simulink model "QPSK_complete2"  (R2016b)
settings: Solver=VariableStepAuto  StartTime=0.0  StopTime=(12+226)*8  RelTol=1e-3  EnableMultiTasking=on
undefined symbols (not defined in the file or in its folder): jsin, K1, K2, rcosine
libraries: dspsigops x2, dspstat3 x1, dspsrcs4 x1, simulink x1
settings Model: Creator=coltmt  LastModifiedBy=colttom
settings OptimizationCC: LifeSpan=inf
settings DebuggingCC: SFUnexpectedBacktrackingDiag=warning  SFNoUnconditionalDefaultTransitionDiag=warning  SFExecutionAtInitializationDiag=none
settings GRTTargetCC: TargetLangStandard=C89/C90 (ANSI)  GeneratePreprocessorConditionals=Disable all
settings ConfigComp: CovMetricSettings=dw  CovHtmlReporting=on  CovSaveCumulativeToWorkspaceVar=on  CovSaveSingleToWorkspaceVar=on  CovExternalEMLEnable=off

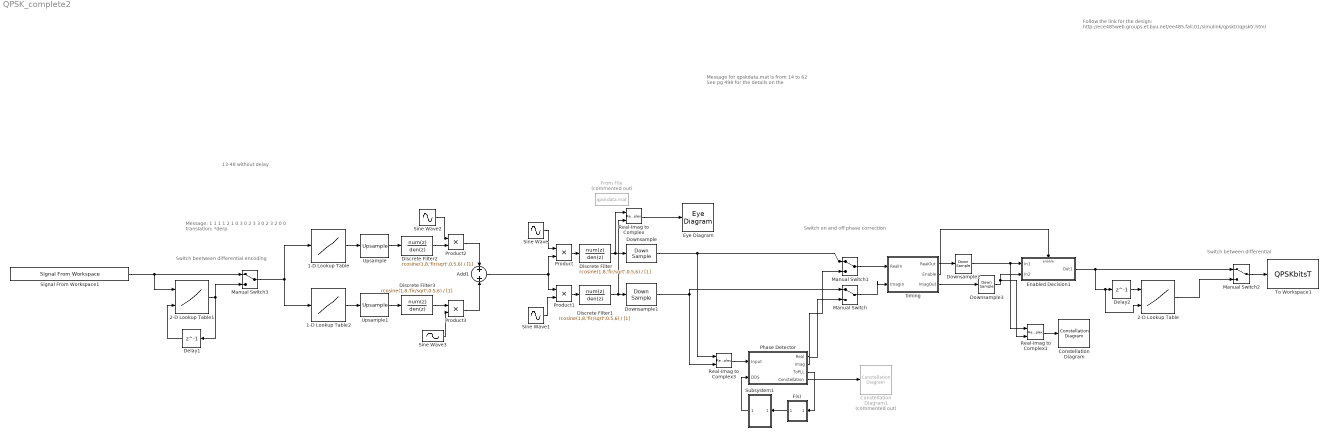
== system QPSK_complete2 ==
  note: Switch beetween differential encoding
  note: Switch between differential
  note: Switch on and off phase correction
  note: 13-48 without delay
  note: Message: 1 1 1 1 2 1 0 3 0 2 3 3 0 2 3 2 0 0
      | translation: *derp
  note: Follow the link for the design: http://ece485web.groups.et.byu.net/ee485.fall.01/simulink/qpsktr/qpsktr.html
  note: Message for qpskdata.mat is from 14 to 62
      |
      | See pg 498 for the details on the
  1-D Lookup Table : Lookup_n-D  NumberOfTableDimensions=1  BreakpointsForDimension1=[0 1 2 3]  Table=[1 -1 1 -1]*3/sqrt(2)  InternalRulePriority=Speed  RndMeth=Simplest  InputSameDT=on
  1-D Lookup Table2 : Lookup_n-D  NumberOfTableDimensions=1  BreakpointsForDimension1=[0 1 2 3]  Table=[1 1 -1 -1]*3/sqrt(2)  InternalRulePriority=Speed  RndMeth=Simplest  InputSameDT=on
  2-D Lookup Table : Lookup_n-D  BreakpointsForDimension1=[0:3]  BreakpointsForDimension2=[0:3]  Table=[0 1 2 3; 2 0 3 1; 1 3 0 2;3 2 1 0]  InternalRulePriority=Speed  RndMeth=Simplest  InputSameDT=on
  2-D Lookup Table1 : Lookup_n-D  BreakpointsForDimension1=[0:3]  BreakpointsForDimension2=[0:3]  Table=[0 1 2 3;1 3 0 2;2 0 3 1;3 2 1 0]  InternalRulePriority=Speed  RndMeth=Simplest  InputSameDT=on
  Add1 : Sum
  Constellation Diagram : ConstellationDiagram
  Constellation Diagram1 : ConstellationDiagram  Commented=on
  Delay1 : Delay  DelayLength=1
  Delay2 : Delay  DelayLength=1
  Discrete Filter{,1..3} (4 alike) : DiscreteFilter  Numerator=rcosine(1,8,'fir/sqrt',0.5,6)  Denominator=[1]
  Downsample : DownSample  N=16/2  InputProcessing=Inherited (this choice will be removed - see release notes)  RateOptions=Allow multirate processing
  Downsample1 : DownSample  N=16/2  InputProcessing=Inherited (this choice will be removed - see release notes)  RateOptions=Allow multirate processing
  Downsample2 : DownSample  RateOptions=Allow multirate processing
  Downsample3 : DownSample  RateOptions=Allow multirate processing
  Enabled Decision1 : Subsystem  TreatAsAtomicUnit=on
  Eye Diagram : EyeDiagram
  F(s) : Subsystem
  From File : FromFile  Commented=on  FileName=qpskdata.mat  SampleTime=1
  Manual Switch{,1..3} (4 alike) : ManualSwitch
  Phase Detector : Subsystem
  Product{,1..3} (4 alike) : Product
  Real-Imag to Complex : RealImagToComplex
  Real-Imag to Complex1 : RealImagToComplex
  Real-Imag to Complex3 : RealImagToComplex
  Signal From Workspace1 : dspsrcs4/Signal From Workspace  X=[1 2 3 0 0 2 3 1 3 2 1 0 3 2 0 2 0 1 4 2 3 1 0 2 3 1 2 3 0 3 2 1 2 3 0 2 3 3 1 2 3 1 2 3 1 2 3 1 2 1 2 1 2 2 1 2 1 2 1 2 1 2 1 2 1 2 1 2 1 2 1 0 0 3 2 0 1 2 0 1 3 2 3 1 1 1 1 1 0 0 0 1 1 0 0 1 1 1 1 2 1 0 3 0 2 3 3 0 2 3 2 0 0]  Ts=8  nsamps=1  OutputAfterFinalValue=Setting to zero  ignoreOrWarnInputAndFrameLengths=off  OutputFrames=off
  Sine Wave : Sin  Amplitude=sqrt(2)  Frequency=2*pi/4  Phase=pi/2  SampleTime=.5
  Sine Wave1 : Sin  Amplitude=-sqrt(2)  Frequency=2*pi/4  SampleTime=.5
  Sine Wave2 : Sin  Amplitude=sqrt(2)  Frequency=2*pi/4  Phase=pi/2  SampleTime=.5
  Sine Wave3 : Sin  Amplitude=-sqrt(2)  Frequency=2*pi/4  SampleTime=.5
  Subsystem1 : Subsystem
  To Workspace1 : ToWorkspace  VariableName=QPSKbitsT  SampleTime=-1
      settings: Save2DSignal=2-D array (concatenate along first dimension)
  Upsample : dspsigops/Upsample  N=16  phase=0  InputProcessing=Inherited (this choice will be removed - see release notes)  RateOptions=Allow multirate processing  ic=0  mode=Unused parameter value
  Upsample1 : dspsigops/Upsample  N=16  phase=0  InputProcessing=Inherited (this choice will be removed - see release notes)  RateOptions=Allow multirate processing  ic=0  mode=Unused parameter value
  timing : Subsystem
  wires:
  Sine Wave1/1 -> Product1/2
  Sine Wave/1 -> Product/1
  Product1/1 -> Discrete Filter1/1
  Product/1 -> Discrete Filter/1
  Discrete Filter/1 -> Downsample/1, Real-Imag to Complex/1
  Discrete Filter1/1 -> Downsample1/1, Real-Imag to Complex/2
  Real-Imag to Complex/1 -> Eye Diagram/1
  Real-Imag to Complex1/1 -> Constellation Diagram/1
  1-D Lookup Table/1 -> Upsample/1
  1-D Lookup Table2/1 -> Upsample1/1
  Upsample/1 -> Discrete Filter2/1
  Upsample1/1 -> Discrete Filter3/1
  Discrete Filter2/1 -> Product2/2
  Sine Wave2/1 -> Product2/1
  Discrete Filter3/1 -> Product3/1
  Sine Wave3/1 -> Product3/2
  Product3/1 -> Add1/2
  Product2/1 -> Add1/1
  Downsample2/1 -> Enabled Decision1/1(In1), Real-Imag to Complex1/1
  Downsample3/1 -> Enabled Decision1/2(In2), Real-Imag to Complex1/2
  Add1/1 -> Product1/1, Product/2
  timing/1(RealOut) -> Downsample2/1
  timing/2(Enable) -> Enabled Decision1/Enable
  timing/3(ImagOut) -> Downsample3/1
  F(s)/1(Out1) -> Subsystem1/1(In1)
  Subsystem1/1(Out1) -> Phase Detector/2(DDS)
  Phase Detector/3(ToPLL) -> F(s)/1(In1)
  Real-Imag to Complex3/1 -> Phase Detector/1(Input)
  Phase Detector/4(Constellation) -> Constellation Diagram1/1
  Downsample/1 -> Manual Switch1/1, Real-Imag to Complex3/1
  Downsample1/1 -> Manual Switch/1, Real-Imag to Complex3/2
  Manual Switch1/1 -> timing/1(RealIn)
  Phase Detector/1(Real) -> Manual Switch1/2
  Manual Switch/1 -> timing/2(ImagIn)
  Phase Detector/2(Imag) -> Manual Switch/2
  Enabled Decision1/1(Out1) -> 2-D Lookup Table/2, Delay2/1, Manual Switch2/1
  2-D Lookup Table/1 -> Manual Switch2/2
  Delay2/1 -> 2-D Lookup Table/1
  Manual Switch2/1 -> To Workspace1/1
  Manual Switch3/1 -> 1-D Lookup Table/1, 1-D Lookup Table2/1
  2-D Lookup Table1/1 -> Delay1/1, Manual Switch3/2
  Delay1/1 -> 2-D Lookup Table1/2
  Signal From Workspace1/1 -> 2-D Lookup Table1/1, Manual Switch3/1

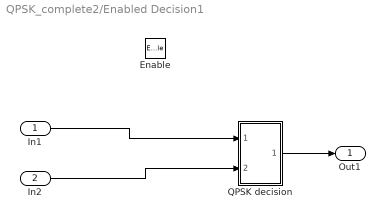
== system QPSK_complete2/Enabled Decision1 ==
  In1 : Inport
  In2 : Inport  Port=2
  Enable : EnablePort
  "QPSK decision " : Subsystem
  Out1 : Outport
  wires:
  "QPSK decision "/1(Out1) -> Out1/1
  In1/1 -> "QPSK decision "/1(In1)
  In2/1 -> "QPSK decision "/2(In2)

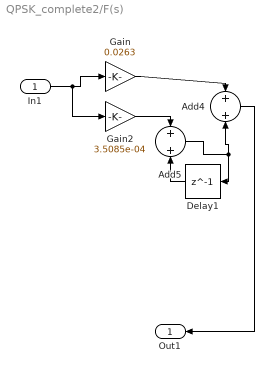
== system QPSK_complete2/F(s) ==
  In1 : Inport
  Add4 : Sum
  Add5 : Sum
  Delay1 : Delay  DelayLength=1
  Gain : Gain  Gain=0.0263
  Gain2 : Gain  Gain=3.5085e-04
  Out1 : Outport
  wires:
  Gain/1 -> Add4/1
  Delay1/1 -> Add5/2
  Add5/1 -> Delay1/1, Add4/2
  Gain2/1 -> Add5/1
  Add4/1 -> Out1/1
  In1/1 -> Gain2/1, Gain/1

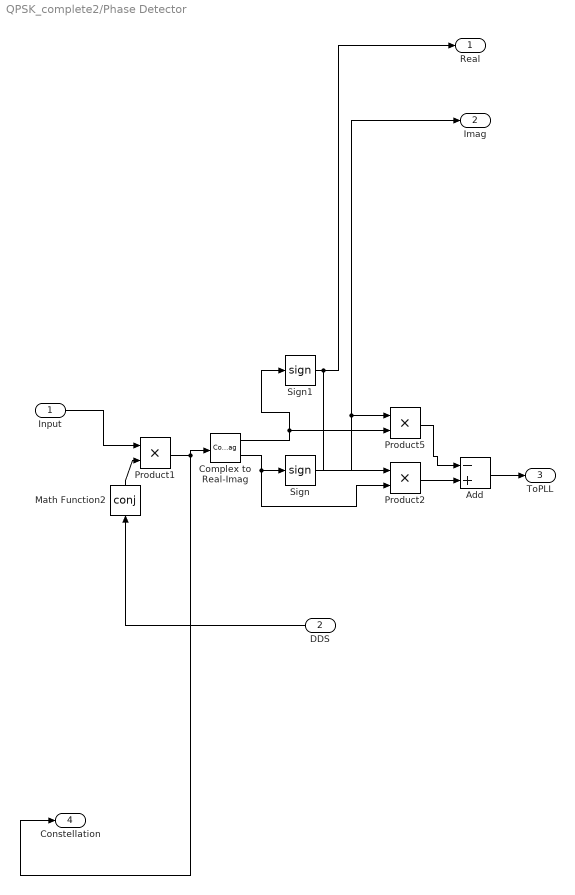
== system QPSK_complete2/Phase Detector ==
  Input : Inport
  DDS : Inport  Port=2
  Add : Sum  Inputs=-+
  Complex to Real-Imag : ComplexToRealImag
  Math Function2 : Math  Operator=conj  SaturateOnIntegerOverflow=on
  Product1 : Product
  Product2 : Product
  Product5 : Product
  Sign : Signum
  Sign1 : Signum
  Real : Outport
  Imag : Outport  Port=2
  ToPLL : Outport  Port=3
  Constellation : Outport  Port=4
  wires:
  Add/1 -> ToPLL/1
  DDS/1 -> Math Function2/1
  Complex to Real-Imag/2 -> Product2/2, Sign/1
  Math Function2/1 -> Product1/2
  Product5/1 -> Add/1
  Product2/1 -> Add/2
  Input/1 -> Product1/1
  Complex to Real-Imag/1 -> Sign1/1, Product5/2
  Sign1/1 -> Real/1, Product2/1
  Sign/1 -> Imag/1, Product5/1
  Product1/1 -> Constellation/1, Complex to Real-Imag/1

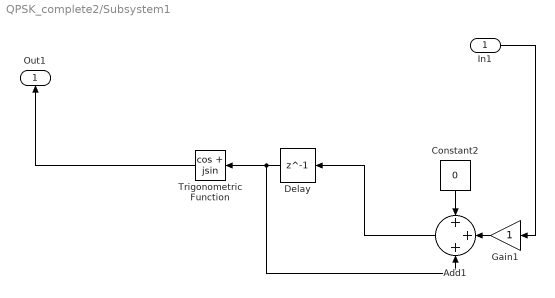
== system QPSK_complete2/Subsystem1 ==
  In1 : Inport
  Add1 : Sum  Inputs=+++
  Constant2 : Constant  Value=0
  Delay : Delay  DelayLength=1
  Gain1 : Gain
  Trigonometric Function : Trigonometry  Operator=cos + jsin
  Out1 : Outport
  wires:
  In1/1 -> Gain1/1
  Constant2/1 -> Add1/1
  Add1/1 -> Delay/1
  Delay/1 -> Trigonometric Function/1, Add1/3
  Gain1/1 -> Add1/2
  Trigonometric Function/1 -> Out1/1

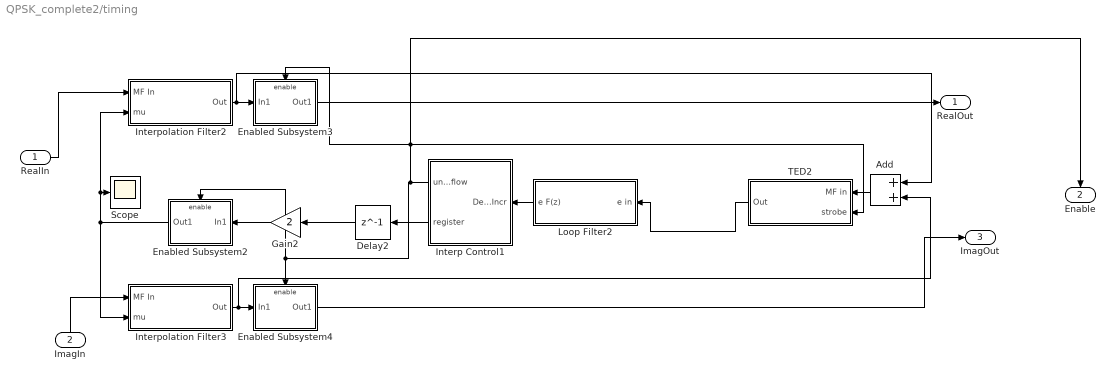
== system QPSK_complete2/timing ==
  RealIn : Inport
  ImagIn : Inport  Port=2
  Add : Sum
  Delay2 : Delay  DelayLength=1
  Enabled Subsystem2 : Subsystem  TreatAsAtomicUnit=on
  Enabled Subsystem3 : Subsystem  TreatAsAtomicUnit=on
  Enabled Subsystem4 : Subsystem  TreatAsAtomicUnit=on
  Gain2 : Gain  Gain=2
  Interp Control1 : Subsystem
  Interpolation Filter2 : Subsystem
  Interpolation Filter3 : Subsystem
  Loop Filter2 : Subsystem
  Scope : Scope
  TED2 : Subsystem
  RealOut : Outport
  Enable : Outport  Port=2
  ImagOut : Outport  Port=3
  wires:
  Interpolation Filter3/1(Out) -> Add/2, Enabled Subsystem4/1(In1)
  Gain2/1 -> Enabled Subsystem2/1(In1)
  Enabled Subsystem4/1(Out1) -> ImagOut/1
  Interpolation Filter2/1(Out) -> Add/1, Enabled Subsystem3/1(In1)
  Enabled Subsystem2/1(Out1) -> Scope/1, Interpolation Filter2/2(mu), Interpolation Filter3/2(mu)
  Delay2/1 -> Gain2/1
  Loop Filter2/1(e F(z)) -> Interp Control1/1(Delta Incr)
  TED2/1(Out) -> Loop Filter2/1(e in)
  RealIn/1 -> Interpolation Filter2/1(MF In)
  ImagIn/1 -> Interpolation Filter3/1(MF In)
  Interp Control1/2(register) -> Delay2/1
  Add/1 -> TED2/1(MF in)
  Interp Control1/1(underflow) -> Enable/1, TED2/2(strobe), Enabled Subsystem3/Enable, Enabled Subsystem4/Enable, Enabled Subsystem2/Enable
  Enabled Subsystem3/1(Out1) -> RealOut/1

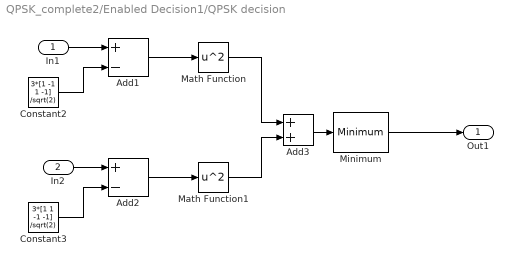
== system QPSK_complete2/Enabled Decision1/QPSK decision  ==
  In1 : Inport
  In2 : Inport  Port=2
  Add1 : Sum  Inputs=+-
  Add2 : Sum  Inputs=+-
  Add3 : Sum
  Constant2 : Constant  Value=3*[1 -1 1 -1] /sqrt(2)
  Constant3 : Constant  Value=3*[1 1 -1 -1] /sqrt(2)
  Math Function : Math  Operator=square  SaturateOnIntegerOverflow=on
  Math Function1 : Math  Operator=square  SaturateOnIntegerOverflow=on
  Minimum : dspstat3/Minimum  operation=minimum  fcn=Index  indexBase=Zero  operateOver=Each column  Dimension=1  InputProcessing=Columns as channels (frame based)  reset=None  roiEnable=off  roiType=Rectangles  roiPortion=Entire ROI  roiOutput=Individual statistics for each ROI  roiFlag=off  roundingMode=Floor  overflowMode=off
  Out1 : Outport
  wires:
  Math Function/1 -> Add3/1
  Math Function1/1 -> Add3/2
  Add3/1 -> Minimum/1
  Minimum/1 -> Out1/1
  Add1/1 -> Math Function/1
  Add2/1 -> Math Function1/1
  Constant3/1 -> Add2/2
  Constant2/1 -> Add1/2
  In1/1 -> Add1/1
  In2/1 -> Add2/1

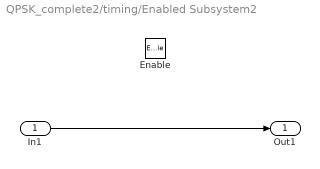
== system QPSK_complete2/timing/Enabled Subsystem2 ==
  In1 : Inport
  Enable : EnablePort
  Out1 : Outport
  wires:
  In1/1 -> Out1/1

== system QPSK_complete2/timing/Enabled Subsystem3 ==
  In1 : Inport
  Enable : EnablePort
  Out1 : Outport
  wires:
  In1/1 -> Out1/1

== system QPSK_complete2/timing/Enabled Subsystem4 ==
  In1 : Inport
  Enable : EnablePort
  Out1 : Outport
  wires:
  In1/1 -> Out1/1

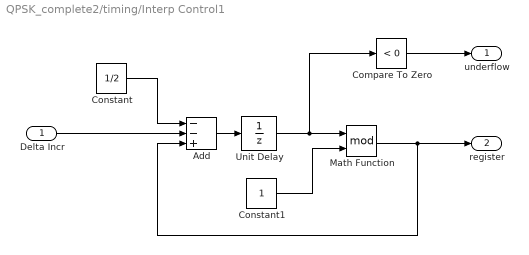
== system QPSK_complete2/timing/Interp Control1 ==
  Delta Incr : Inport
  Add : Sum  Inputs=--+
  Compare To Zero : simulink/Logic and Bit Operations/Compare To Zero  relop=<  OutDataTypeStr=boolean
  Constant : Constant  Value=1/2
  Constant1 : Constant
  Math Function : Math  Operator=mod  SaturateOnIntegerOverflow=on
  Unit Delay : UnitDelay  SampleTime=-1
  underflow : Outport
  register : Outport  Port=2
  wires:
  Delta Incr/1 -> Add/2
  Constant/1 -> Add/1
  Add/1 -> Unit Delay/1
  Constant1/1 -> Math Function/2
  Unit Delay/1 -> Compare To Zero/1, Math Function/1
  Math Function/1 -> Add/3, register/1
  Compare To Zero/1 -> underflow/1

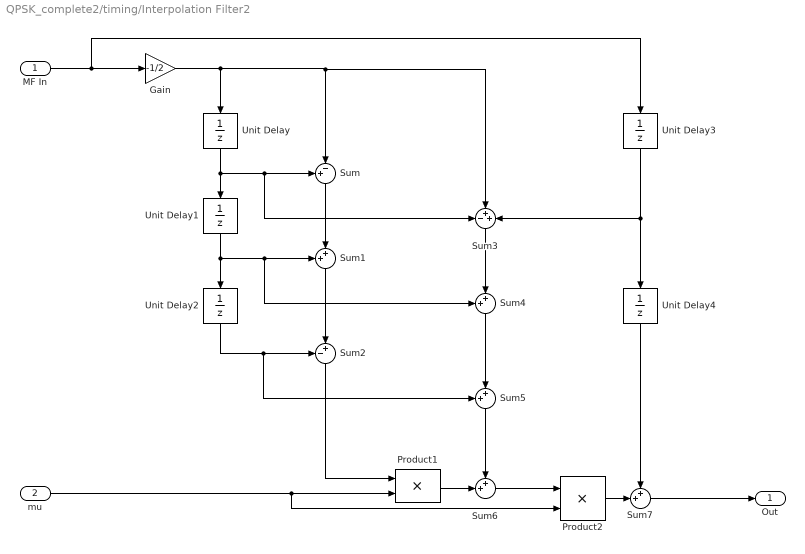
== system QPSK_complete2/timing/Interpolation Filter2 ==
  MF In : Inport
  mu : Inport  Port=2
  Gain : Gain  Gain=-1/2
  Product1 : Product  SaturateOnIntegerOverflow=on  InputSameDT=on  OutDataTypeStr=Inherit: Same as first input
  Product2 : Product  SaturateOnIntegerOverflow=on  InputSameDT=on  OutDataTypeStr=Inherit: Same as first input
  Sum : Sum  Inputs=+-|  SaturateOnIntegerOverflow=on  InputSameDT=on  OutDataTypeStr=Inherit: Same as first input
  Sum{1,4..7} (5 alike) : Sum  Inputs=++|  SaturateOnIntegerOverflow=on  InputSameDT=on  OutDataTypeStr=Inherit: Same as first input
  Sum2 : Sum  Inputs=-+|  SaturateOnIntegerOverflow=on  InputSameDT=on  OutDataTypeStr=Inherit: Same as first input
  Sum3 : Sum  Inputs=-++  SaturateOnIntegerOverflow=on  InputSameDT=on  OutDataTypeStr=Inherit: Same as first input
  Unit Delay{,1..4} (5 alike) : UnitDelay  SampleTime=-1
  Out : Outport
  wires:
  Sum1/1 -> Sum2/2
  Sum/1 -> Sum1/2
  Unit Delay/1 -> Sum3/1, Sum/1, Unit Delay1/1
  Unit Delay1/1 -> Sum4/1, Sum1/1, Unit Delay2/1
  Unit Delay2/1 -> Sum5/1, Sum2/1
  Sum5/1 -> Sum6/1
  Product1/1 -> Sum6/2
  Sum4/1 -> Sum5/2
  Sum3/1 -> Sum4/2
  MF In/1 -> Unit Delay3/1, Gain/1
  Gain/1 -> Unit Delay/1, Sum/2, Sum3/2
  Product2/1 -> Sum7/2
  Unit Delay4/1 -> Sum7/1
  Sum6/1 -> Product2/1
  Sum7/1 -> Out/1
  Unit Delay3/1 -> Sum3/3, Unit Delay4/1
  Sum2/1 -> Product1/1
  mu/1 -> Product2/2, Product1/2

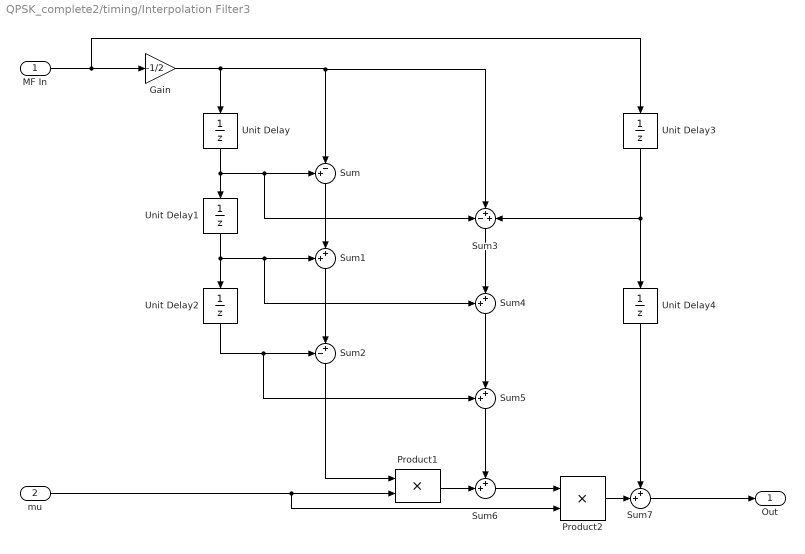
== system QPSK_complete2/timing/Interpolation Filter3 ==
  MF In : Inport
  mu : Inport  Port=2
  Gain : Gain  Gain=-1/2
  Product1 : Product  SaturateOnIntegerOverflow=on  InputSameDT=on  OutDataTypeStr=Inherit: Same as first input
  Product2 : Product  SaturateOnIntegerOverflow=on  InputSameDT=on  OutDataTypeStr=Inherit: Same as first input
  Sum : Sum  Inputs=+-|  SaturateOnIntegerOverflow=on  InputSameDT=on  OutDataTypeStr=Inherit: Same as first input
  Sum{1,4..7} (5 alike) : Sum  Inputs=++|  SaturateOnIntegerOverflow=on  InputSameDT=on  OutDataTypeStr=Inherit: Same as first input
  Sum2 : Sum  Inputs=-+|  SaturateOnIntegerOverflow=on  InputSameDT=on  OutDataTypeStr=Inherit: Same as first input
  Sum3 : Sum  Inputs=-++  SaturateOnIntegerOverflow=on  InputSameDT=on  OutDataTypeStr=Inherit: Same as first input
  Unit Delay{,1..4} (5 alike) : UnitDelay  SampleTime=-1
  Out : Outport
  wires:
  Sum1/1 -> Sum2/2
  Sum/1 -> Sum1/2
  Unit Delay/1 -> Sum3/1, Sum/1, Unit Delay1/1
  Unit Delay1/1 -> Sum4/1, Sum1/1, Unit Delay2/1
  Unit Delay2/1 -> Sum5/1, Sum2/1
  Sum5/1 -> Sum6/1
  Product1/1 -> Sum6/2
  Sum4/1 -> Sum5/2
  Sum3/1 -> Sum4/2
  MF In/1 -> Unit Delay3/1, Gain/1
  Gain/1 -> Unit Delay/1, Sum/2, Sum3/2
  Product2/1 -> Sum7/2
  Unit Delay4/1 -> Sum7/1
  Sum6/1 -> Product2/1
  Sum7/1 -> Out/1
  Unit Delay3/1 -> Sum3/3, Unit Delay4/1
  Sum2/1 -> Product1/1
  mu/1 -> Product2/2, Product1/2

== system QPSK_complete2/timing/Loop Filter2 ==
  e in : Inport
  Discrete Filter : DiscreteFilter  Numerator=[(K1+K2) -K1]  Denominator=[1 -1]
  e F(z) : Outport
  wires:
  e in/1 -> Discrete Filter/1
  Discrete Filter/1 -> e F(z)/1

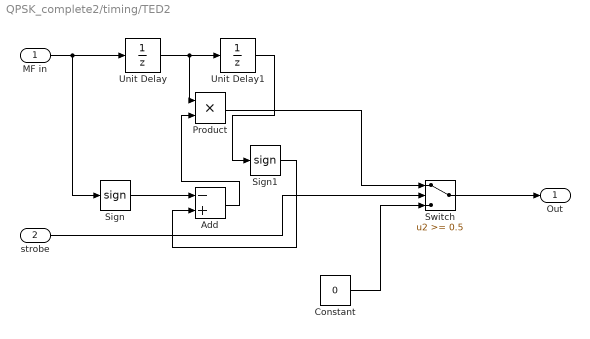
== system QPSK_complete2/timing/TED2 ==
  MF in : Inport
  strobe : Inport  Port=2
  Add : Sum  Inputs=-+
  Constant : Constant  Value=0
  Product : Product
  Sign : Signum
  Sign1 : Signum
  Switch : Switch  Threshold=0.5  SaturateOnIntegerOverflow=on
  Unit Delay : UnitDelay  SampleTime=-1
  Unit Delay1 : UnitDelay  SampleTime=-1
  Out : Outport
  wires:
  Switch/1 -> Out/1
  Constant/1 -> Switch/3
  strobe/1 -> Switch/2
  MF in/1 -> Sign/1, Unit Delay/1
  Unit Delay/1 -> Product/1, Unit Delay1/1
  Sign/1 -> Add/1
  Add/1 -> Product/2
  Unit Delay1/1 -> Sign1/1
  Sign1/1 -> Add/2
  Product/1 -> Switch/1
